simulink library "csu_ftc_final_thruster_cmd_lib"  (R2014b)
settings: Solver=ode45  StartTime=0.0  StopTime=10.0  RelTol=1e-3
values from neighbouring files (symbols this model uses):
  act_full_on_duration = uint32( 120 )    [csc_act_actuator_manager_init.m]
  fsw_dt = 0.1    [csu_taf_thruster_arm_fire_test.m]
undefined symbols (not defined in the file or in its folder): coarse10_time, coarse11_time, coarse12_time, coarse1_time, coarse2_time, coarse3_time, coarse4_time, coarse5_time, coarse6_time, coarse7_time, coarse8_time, coarse9_time, fine10_time, fine11_time, fine12_time, fine1_time, fine2_time, fine3_time, fine4_time, fine5_time, fine6_time, fine7_time, fine8_time, fine9_time, main_biprop_monoprop, main_thruster_cmd
libraries: simulink x8, util_event_lib x8, util_info_lib x1, csu_tts_thruster_time_safety_lib x1
settings Model: Creator=escrane  LastModifiedBy=mstewart

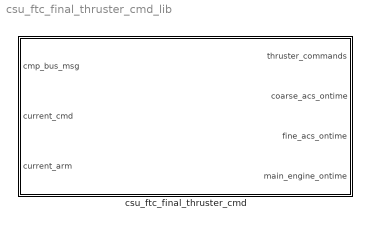
== system csu_ftc_final_thruster_cmd_lib ==
  " csu_ftc_final_thruster_cmd" : Subsystem

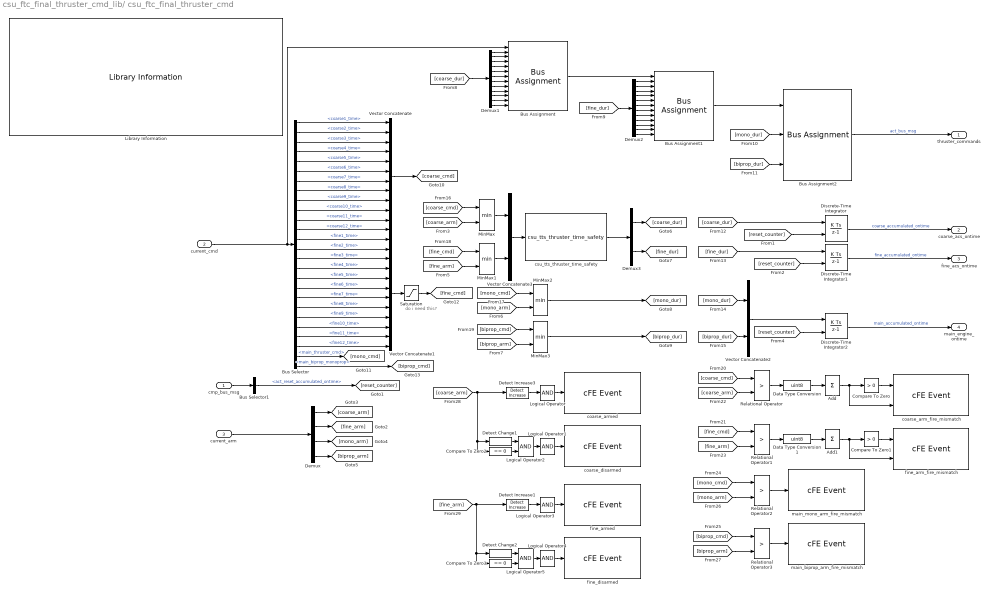
== system csu_ftc_final_thruster_cmd_lib/ csu_ftc_final_thruster_cmd ==
  note: do i need this?
  cmp_bus_msg : Inport
  current_cmd : Inport  Port=2
  current_arm : Inport  Port=3
  Add : Sum  Inputs=+
  Add1 : Sum  Inputs=+
  Bus Assignment : BusAssignment  AssignedSignals=coarse1_time,coarse2_time,coarse3_time,coarse4_time,coarse5_time,coarse6_time,coarse7_time,coarse8_time,coarse9_time,coarse10_time,coarse11_time,coarse12_time
  Bus Assignment1 : BusAssignment  AssignedSignals=fine1_time,fine2_time,fine3_time,fine4_time,fine5_time,fine6_time,fine7_time,fine8_time,fine9_time,fine10_time,fine11_time,fine12_time
  Bus Assignment2 : BusAssignment  AssignedSignals=main_thruster_cmd,main_biprop_monoprop
  Bus Selector : BusSelector  OutputSignals=coarse1_time,coarse2_time,coarse3_time,coarse4_time,coarse5_time,coarse6_time,coarse7_time,coarse8_time,coarse9_time,coarse10_time,coarse11_time,coarse12_time,fine1_time,fine2_time,fine3_time,fine4_time,fine5_time,fine6_time,fine7_time,fine8_time,fine9_time,fine10_time,fine11_time,fine12_time,main_thruster_cmd,main_biprop_monoprop
  Bus Selector1 : BusSelector  OutputSignals=act_reset_accumulated_ontime
  Compare To Zero : simulink/Logic and Bit Operations/Compare To Zero  relop=>  OutDataTypeStr=boolean
  Compare To Zero1 : simulink/Logic and Bit Operations/Compare To Zero  relop=>  OutDataTypeStr=boolean
  Compare To Zero2 : simulink/Logic and Bit Operations/Compare To Zero  relop===  OutDataTypeStr=boolean
  Compare To Zero3 : simulink/Logic and Bit Operations/Compare To Zero  relop===  OutDataTypeStr=boolean
  Data Type Conversion : DataTypeConversion  OutDataTypeStr=uint8
  Data Type Conversion1 : DataTypeConversion  OutDataTypeStr=uint8
  Demux : Demux  Outputs=[12 12 1 1]
  Demux1 : Demux  Outputs=12
  Demux2 : Demux  Outputs=12
  Demux3 : Demux  Outputs=[12 12]
  Detect Change1 : simulink/Logic and Bit Operations/Detect Change  vinit=0  InputProcessing=Inherited  OutDataTypeStr=boolean
  Detect Change2 : simulink/Logic and Bit Operations/Detect Change  vinit=0  InputProcessing=Inherited  OutDataTypeStr=boolean
  Detect Increase1 : simulink/Logic and Bit Operations/Detect Increase  vinit=0.0  InputProcessing=Inherited  OutDataTypeStr=boolean
  Detect Increase3 : simulink/Logic and Bit Operations/Detect Increase  vinit=0.0  InputProcessing=Inherited  OutDataTypeStr=boolean
  Discrete-Time Integrator : DiscreteIntegrator  gainval=1/fsw_dt  ExternalReset=rising  InitialConditionSetting=Compatibility  SampleTime=-1  OutDataTypeStr=uint32
  Discrete-Time Integrator1 : DiscreteIntegrator  gainval=1/fsw_dt  ExternalReset=rising  InitialConditionSetting=Compatibility  SampleTime=-1  OutDataTypeStr=uint32
  Discrete-Time Integrator2 : DiscreteIntegrator  gainval=1/fsw_dt  ExternalReset=rising  InitialConditionSetting=Compatibility  SampleTime=-1  OutDataTypeStr=uint32
  Library Information : util_info_lib/Library Information  owner='escrane'
  Logical Operator{,1,3..4} (4 alike) : Logic  Inputs=1  AllPortsSameDT=off  OutDataTypeStr=boolean
  Logical Operator2 : Logic  AllPortsSameDT=off  OutDataTypeStr=boolean
  Logical Operator5 : Logic  AllPortsSameDT=off  OutDataTypeStr=boolean
  MinMax{,1..3} (4 alike) : MinMax  Inputs=2  OutDataTypeStr=uint8
  Relational Operator{,1..3} (4 alike) : RelationalOperator  Operator=>
  Saturation : Saturate  UpperLimit=act_full_on_duration  LowerLimit=0
  Vector Concatenate : Concatenate  NumInputs=12
  Vector Concatenate1 : Concatenate  NumInputs=12
  Vector Concatenate2 : Concatenate
  Vector Concatenate3 : Concatenate
  coarse_arm_fire_mismatch : util_event_lib/cFE Event  event_message='Coarse ACS commanded longer than enabled: %u thrusters'  event_id=19  event_severity=ERROR  event_use_enums=off  event_enum_types={}
  coarse_armed : util_event_lib/cFE Event  event_message='Coarse thrusters enabled'  event_id=26  event_severity=INFORMATION  event_use_enums=off  event_enum_types={}
  coarse_disarmed : util_event_lib/cFE Event  event_message='Coarse thrusters disabled'  event_id=26  event_severity=INFORMATION  event_use_enums=off  event_enum_types={}
  csu_tts_thruster_time_safety : csu_tts_thruster_time_safety_lib/csu_tts_thruster_time_safety
  fine_arm_fire_mismatch : util_event_lib/cFE Event  event_message='Fine ACS commanded longer than enabled: %u thrusters'  event_id=20  event_severity=ERROR  event_use_enums=off  event_enum_types={}
  fine_armed : util_event_lib/cFE Event  event_message='Fine thrusters enabled'  event_id=26  event_severity=INFORMATION  event_use_enums=off  event_enum_types={}
  fine_disarmed : util_event_lib/cFE Event  event_message='Fine thrusters disabled'  event_id=26  event_severity=INFORMATION  event_use_enums=off  event_enum_types={}
  main_biprop_arm_fire_mismatch : util_event_lib/cFE Event  event_message='Biprop main valve commanded longer than enabled'  event_id=23  event_severity=ERROR  event_use_enums=off  event_enum_types={}
  main_mono_arm_fire_mismatch : util_event_lib/cFE Event  event_message='Monoprop main valve commanded longer than enabled'  event_id=22  event_severity=ERROR  event_use_enums=off  event_enum_types={}
  thruster_commands : Outport
  coarse_acs_ontime : Outport  Port=2
  fine_acs_ontime : Outport  Port=3
  main_engine_ontime : Outport  Port=4
  wires:
  Logical Operator5/1 -> Logical Operator4/1
  Compare To Zero3/1 -> Logical Operator5/2
  Detect Change2/1 -> Logical Operator5/1
  Logical Operator4/1 -> fine_disarmed/1
  Logical Operator3/1 -> fine_armed/1
  Detect Increase1/1 -> Logical Operator3/1
  [fine_arm] -> Compare To Zero3/1, Detect Change2/1, Detect Increase1/1
  Logical Operator2/1 -> Logical Operator1/1
  Compare To Zero2/1 -> Logical Operator2/2
  Detect Change1/1 -> Logical Operator2/1
  Logical Operator1/1 -> coarse_disarmed/1
  Logical Operator/1 -> coarse_armed/1
  Detect Increase3/1 -> Logical Operator/1
  [coarse_arm] -> Detect Increase3/1, Detect Change1/1, Compare To Zero2/1
  Saturation/1 -> [fine_cmd]
  Relational Operator3/1 -> main_biprop_arm_fire_mismatch/1
  Relational Operator2/1 -> main_mono_arm_fire_mismatch/1
  [biprop_cmd] -> Relational Operator3/1
  [mono_cmd] -> Relational Operator2/1
  [biprop_arm] -> Relational Operator3/2
  [mono_arm] -> Relational Operator2/2
  Relational Operator1/1 -> Data Type Conversion1/1
  Compare To Zero1/1 -> fine_arm_fire_mismatch/1
  Add1/1 -> Compare To Zero1/1, fine_arm_fire_mismatch/2
  Data Type Conversion1/1 -> Add1/1
  Compare To Zero/1 -> coarse_arm_fire_mismatch/1
  Add/1 -> Compare To Zero/1, coarse_arm_fire_mismatch/2
  Data Type Conversion/1 -> Add/1
  Relational Operator/1 -> Data Type Conversion/1
  [fine_arm] -> Relational Operator1/2
  [fine_cmd] -> Relational Operator1/1
  [coarse_arm] -> Relational Operator/2
  [coarse_cmd] -> Relational Operator/1
  [biprop_cmd] -> MinMax3/1
  [mono_cmd] -> MinMax2/1
  [fine_cmd] -> MinMax1/1
  [coarse_cmd] -> MinMax/1
  Vector Concatenate1/1 -> Saturation/1
  Vector Concatenate/1 -> [coarse_cmd]
  Bus Selector/26 -> [biprop_cmd]  "<main_biprop_monoprop>"
  Bus Selector/25 -> [mono_cmd]  "<main_thruster_cmd>"
  [biprop_dur] -> Vector Concatenate2/2
  [mono_dur] -> Vector Concatenate2/1
  [fine_dur] -> Discrete-Time Integrator1/1
  [coarse_dur] -> Discrete-Time Integrator/1
  MinMax3/1 -> [biprop_dur]
  MinMax2/1 -> [mono_dur]
  Demux3/2 -> [fine_dur]
  csu_tts_thruster_time_safety/1 -> Demux3/1
  Vector Concatenate3/1 -> csu_tts_thruster_time_safety/1
  MinMax1/1 -> Vector Concatenate3/2
  Demux3/1 -> [coarse_dur]
  [biprop_dur] -> Bus Assignment2/3
  [mono_dur] -> Bus Assignment2/2
  [fine_dur] -> Demux2/1
  [coarse_dur] -> Demux1/1
  MinMax/1 -> Vector Concatenate3/1
  Bus Assignment2/1 -> thruster_commands/1  "act_bus_msg"
  Bus Assignment1/1 -> Bus Assignment2/1
  Bus Assignment/1 -> Bus Assignment1/1
  Demux2/1 -> Bus Assignment1/2
  Demux2/12 -> Bus Assignment1/13
  Demux2/2 -> Bus Assignment1/3
  Demux2/6 -> Bus Assignment1/7
  Demux2/8 -> Bus Assignment1/9
  Demux2/3 -> Bus Assignment1/4
  Demux2/7 -> Bus Assignment1/8
  Demux2/5 -> Bus Assignment1/6
  Demux2/9 -> Bus Assignment1/10
  Demux2/10 -> Bus Assignment1/11
  Demux2/11 -> Bus Assignment1/12
  Demux2/4 -> Bus Assignment1/5
  Demux1/1 -> Bus Assignment/2
  Demux1/12 -> Bus Assignment/13
  Demux1/2 -> Bus Assignment/3
  Demux1/6 -> Bus Assignment/7
  Demux1/8 -> Bus Assignment/9
  Demux1/3 -> Bus Assignment/4
  Demux1/7 -> Bus Assignment/8
  Demux1/5 -> Bus Assignment/6
  Demux1/9 -> Bus Assignment/10
  Demux1/10 -> Bus Assignment/11
  Demux1/11 -> Bus Assignment/12
  Demux1/4 -> Bus Assignment/5
  [biprop_arm] -> MinMax3/2
  [mono_arm] -> MinMax2/2
  [fine_arm] -> MinMax1/2
  Demux/4 -> [biprop_arm]
  Demux/3 -> [mono_arm]
  Demux/2 -> [fine_arm]
  Demux/1 -> [coarse_arm]
  current_arm/1 -> Demux/1
  [coarse_arm] -> MinMax/2
  Discrete-Time Integrator2/1 -> main_engine_ontime/1  "main_accumulated_ontime"
  Vector Concatenate2/1 -> Discrete-Time Integrator2/1
  [reset_counter] -> Discrete-Time Integrator2/2
  Bus Selector1/1 -> [reset_counter]  "<act_reset_accumulated_ontime>"
  cmp_bus_msg/1 -> Bus Selector1/1
  Discrete-Time Integrator1/1 -> fine_acs_ontime/1  "fine_accumulated_ontime"
  Discrete-Time Integrator/1 -> coarse_acs_ontime/1  "coarse_accumulated_ontime"
  [reset_counter] -> Discrete-Time Integrator1/2
  [reset_counter] -> Discrete-Time Integrator/2
  Bus Selector/15 -> Vector Concatenate1/3  "<fine3_time>"
  Bus Selector/19 -> Vector Concatenate1/7  "<fine7_time>"
  Bus Selector/18 -> Vector Concatenate1/6  "<fine6_time>"
  Bus Selector/20 -> Vector Concatenate1/8  "<fine8_time>"
  Bus Selector/24 -> Vector Concatenate1/12  "<fine12_time>"
  Bus Selector/22 -> Vector Concatenate1/10  "<fine10_time>"
  Bus Selector/17 -> Vector Concatenate1/5  "<fine5_time>"
  Bus Selector/23 -> Vector Concatenate1/11  "<fine11_time>"
  Bus Selector/16 -> Vector Concatenate1/4  "<fine4_time>"
  Bus Selector/13 -> Vector Concatenate1/1  "<fine1_time>"
  Bus Selector/14 -> Vector Concatenate1/2  "<fine2_time>"
  Bus Selector/21 -> Vector Concatenate1/9  "<fine9_time>"
  Bus Selector/2 -> Vector Concatenate/2  "<coarse2_time>"
  Bus Selector/5 -> Vector Concatenate/5  "<coarse5_time>"
  Bus Selector/9 -> Vector Concatenate/9  "<coarse9_time>"
  Bus Selector/4 -> Vector Concatenate/4  "<coarse4_time>"
  Bus Selector/7 -> Vector Concatenate/7  "<coarse7_time>"
  Bus Selector/8 -> Vector Concatenate/8  "<coarse8_time>"
  Bus Selector/3 -> Vector Concatenate/3  "<coarse3_time>"
  Bus Selector/12 -> Vector Concatenate/12  "<coarse12_time>"
  Bus Selector/11 -> Vector Concatenate/11  "<coarse11_time>"
  Bus Selector/6 -> Vector Concatenate/6  "<coarse6_time>"
  Bus Selector/10 -> Vector Concatenate/10  "<coarse10_time>"
  Bus Selector/1 -> Vector Concatenate/1  "<coarse1_time>"
  current_cmd/1 -> Bus Selector/1, Bus Assignment/1
